simulink model "HaloSim"  (R2019b)
settings: Solver=ode45  StartTime=0.0  StopTime=simTime  FixedStep=10^-5  RelTol=1e-4
values from neighbouring files (symbols this model uses):
  a = zeros(2,1)    [init.m]
  b = zeros(2,1)    [init.m]
  c = zeros(2,1)    [init.m]
  disturbance = 1    [init.m]
  emulation = delta    (= 0.1)    [init.m]
  Gsc = 1.3608    [init.m]
  h = zeros(2,1)    [init.m]
  K = place(A,G,pole)    [init.m]
  k = 0.1    [init.m]
  L2 = 1.1556    [init.m]
  mu = 0.012149    [init.m]
  Omega = 1.8636    [init.m]
  Omega_z = Omega    (= 1.8636)    [init.m]
  phi = 0    [init.m]
  satValue = inf    [init.m]
  sped = 300000    [init.m]
  srp = 1    [init.m]
  x0 = Seq + [ho1;diffho1]    [init.m]
  zeta = 0.9252    [init.m]
libraries: sdolib x1
settings Model: Creator=mohd-  LastModifiedBy=mohd-

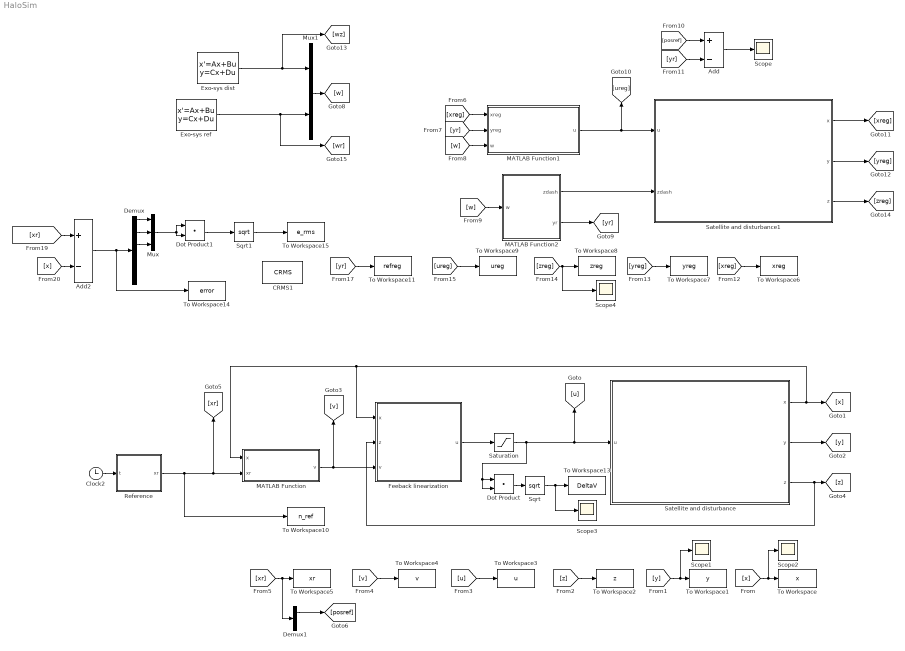
== system HaloSim ==
  Add : Sum  Inputs=+-
  Add2 : Sum  Inputs=+-
  CRMS1 : sdolib/RMS Blocks/CRMS
      settings: SourceProductName=Simulink Design Optimization  SourceProductBaseCode=SO
  Clock2 : Clock
  Demux : Demux  Outputs=6
  Demux1 : Demux  Outputs=[3 3]
  Dot Product : DotProduct  InputSameDT=on  OutDataTypeStr=Inherit: Inherit via internal rule
  Dot Product1 : DotProduct  InputSameDT=on  OutDataTypeStr=Inherit: Inherit via internal rule
  Exo-sys dist : StateSpace  A=[0 -1;1 0]  B=[0;0]  C=eye(2)  D=zeros(2,1)  InitialCondition=[1;0]
  "Exo-sys ref " : StateSpace  A=[0 -Omega;Omega 0]  B=[0;0]  C=eye(2)  D=zeros(2,1)  InitialCondition=[1;0]
  Feeback linearization : MATLAB Function  TreatAsAtomicUnit=on  SystemSampleTime=emulation
  MATLAB Function : MATLAB Function  TreatAsAtomicUnit=on  SystemSampleTime=emulation
  MATLAB Function1 : MATLAB Function  TreatAsAtomicUnit=on  SystemSampleTime=emulation
  MATLAB Function2 : MATLAB Function  TreatAsAtomicUnit=on
  Mux : Mux  Inputs=3
  Mux1 : Mux  Inputs=2
  Reference : MATLAB Function  TreatAsAtomicUnit=on
  Satellite and disturbance : Subsystem
  Satellite and disturbance1 : Subsystem
  Saturation : Saturate  UpperLimit=satValue  LowerLimit=-satValue
  Scope{,1..4} (5 alike) : Scope
  Sqrt : Sqrt  SaturateOnIntegerOverflow=on
  Sqrt1 : Sqrt  SaturateOnIntegerOverflow=on
  To Workspace : ToWorkspace  VariableName=x  SampleTime=10^-3
  To Workspace1 : ToWorkspace  VariableName=y  SampleTime=10^-3
  To Workspace10 : ToWorkspace  VariableName=n_ref  SampleTime=10^-3
  To Workspace11 : ToWorkspace  VariableName=refreg  SampleTime=10^-3
  To Workspace13 : ToWorkspace  VariableName=DeltaV  SampleTime=10^-3
  To Workspace14 : ToWorkspace  VariableName=error  SampleTime=10^-3
  To Workspace15 : ToWorkspace  VariableName=e_rms  SampleTime=10^-3
  To Workspace2 : ToWorkspace  VariableName=z  SampleTime=10^-3
  To Workspace3 : ToWorkspace  VariableName=u  SampleTime=10^-3
  To Workspace4 : ToWorkspace  VariableName=v  SampleTime=10^-3
  To Workspace5 : ToWorkspace  VariableName=xr  SampleTime=10^-3
  To Workspace6 : ToWorkspace  VariableName=xreg  SampleTime=10^-3
  To Workspace7 : ToWorkspace  VariableName=yreg  SampleTime=10^-3
  To Workspace8 : ToWorkspace  VariableName=zreg  SampleTime=10^-3
  To Workspace9 : ToWorkspace  VariableName=ureg  SampleTime=10^-3
  wires:
  Clock2/1 -> Reference/1(t)
  Satellite and disturbance/1(x) -> Feeback linearization/1(x), MATLAB Function/1(x), [x]
  Satellite and disturbance/2(y) -> [y]
  Satellite and disturbance/3(z) -> Feeback linearization/2(z), [z]
  MATLAB Function/1(v) -> Feeback linearization/3(v), [v]
  Reference/1(xr) -> To Workspace10/1, [xr], MATLAB Function/2(xr)
  [x] -> Scope2/1, To Workspace/1
  [y] -> Scope1/1, To Workspace1/1
  [z] -> To Workspace2/1
  [u] -> To Workspace3/1
  [v] -> To Workspace4/1
  [xr] -> Demux1/1, To Workspace5/1
  [xreg] -> MATLAB Function1/1(xreg)
  [yr] -> MATLAB Function1/2(yreg)
  [w] -> MATLAB Function1/3(w)
  [w] -> MATLAB Function2/1(w)
  MATLAB Function2/1(zdash) -> Satellite and disturbance1/2("zdash ")
  MATLAB Function2/2(yr) -> [yr]
  [posref] -> Add/1
  [yr] -> Add/2
  Add/1 -> Scope/1
  [yr] -> To Workspace11/1
  MATLAB Function1/1(u) -> Satellite and disturbance1/1(u), [ureg]
  [yreg] -> To Workspace7/1
  [xreg] -> To Workspace6/1
  Satellite and disturbance1/2(y) -> [yreg]
  Satellite and disturbance1/1(x) -> [xreg]
  Satellite and disturbance1/3(z) -> [zreg]
  [ureg] -> To Workspace9/1
  [zreg] -> Scope4/1, To Workspace8/1
  Add2/1 -> To Workspace14/1, Demux/1
  [xr] -> Add2/1
  Demux/2 -> Mux/2
  [x] -> Add2/2
  Demux/1 -> Mux/1
  Mux/1 -> Dot Product1/1, Dot Product1/2
  Demux/3 -> Mux/3
  Dot Product/1 -> Sqrt/1
  Feeback linearization/1(u) -> Saturation/1
  Saturation/1 -> Dot Product/2, Dot Product/1, Satellite and disturbance/1(u), [u]
  Sqrt/1 -> To Workspace13/1, Scope3/1
  Dot Product1/1 -> Sqrt1/1
  Sqrt1/1 -> To Workspace15/1
  Demux1/1 -> [posref]
  "Exo-sys ref "/1 -> [wr], Mux1/2
  Exo-sys dist/1 -> [wz], Mux1/1
  Mux1/1 -> [w]

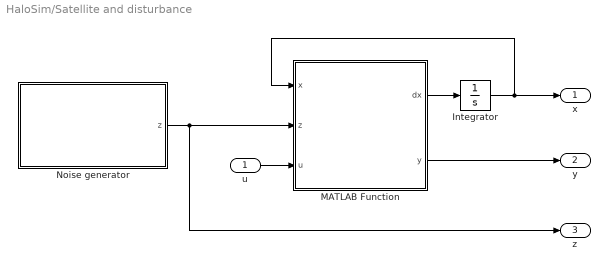
== system HaloSim/Satellite and disturbance ==
  u : Inport
  Integrator : Integrator  InitialCondition=x0
  MATLAB Function : MATLAB Function  TreatAsAtomicUnit=on
  Noise generator : Subsystem
  x : Outport
  y : Outport  Port=2
  z : Outport  Port=3
  wires:
  Integrator/1 -> x/1, MATLAB Function/1(x)
  MATLAB Function/1(dx) -> Integrator/1
  MATLAB Function/2(y) -> y/1
  Noise generator/1(z) -> z/1, MATLAB Function/2(z)
  u/1 -> MATLAB Function/3(u)

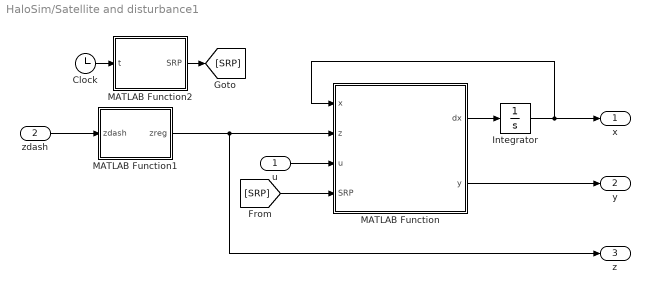
== system HaloSim/Satellite and disturbance1 ==
  u : Inport
  "zdash " : Inport  Port=2
  Clock : Clock
  Integrator : Integrator  InitialCondition=x0
  MATLAB Function : MATLAB Function  TreatAsAtomicUnit=on
  MATLAB Function1 : MATLAB Function  TreatAsAtomicUnit=on
  MATLAB Function2 : MATLAB Function  TreatAsAtomicUnit=on
  x : Outport
  y : Outport  Port=2
  z : Outport  Port=3
  wires:
  Integrator/1 -> x/1, MATLAB Function/1(x)
  MATLAB Function/1(dx) -> Integrator/1
  MATLAB Function/2(y) -> y/1
  "zdash "/1 -> MATLAB Function1/1(zdash)
  u/1 -> MATLAB Function/3(u)
  MATLAB Function1/1(zreg) -> z/1, MATLAB Function/2(z)
  Clock/1 -> MATLAB Function2/1(t)
  MATLAB Function2/1(SRP) -> [SRP]
  [SRP] -> MATLAB Function/4(SRP)

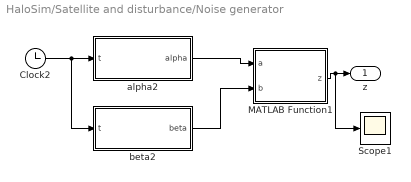
== system HaloSim/Satellite and disturbance/Noise generator ==
  Clock2 : Clock
  MATLAB Function1 : MATLAB Function  TreatAsAtomicUnit=on
  Scope1 : Scope
  alpha2 : MATLAB Function  TreatAsAtomicUnit=on
  beta2 : MATLAB Function  TreatAsAtomicUnit=on
  z : Outport
  wires:
  MATLAB Function1/1(z) -> Scope1/1, z/1
  alpha2/1(alpha) -> MATLAB Function1/1(a)
  beta2/1(beta) -> MATLAB Function1/2(b)
  Clock2/1 -> beta2/1(t), alpha2/1(t)

== matlab function HaloSim/Feeback linearization ==
  data: x input; z input; u output; v input; mu parameter
function u = compensator(x,z,v,mu)
%#codegen


x1 = x(1:3);
x2 = x(4:6);

% M = [-1 0 0;
%     0 -1 0;
%     0 0 0];
% 
% N = [0 -1 0;
%     1 0 0;
%     0 0 0];
% 
% d1r = [-mu - z(4)/(1-mu);0;0];
% d2r = [1-mu + z(4)/mu;0;0];
% 
% ed1 = x1 - d1r;
% absed1 = sqrt(ed1(1)^2+ed1(2)^2+ed1(3)^2);
% ed2 = x1 - d2r;
% absed2 = sqrt(ed2(1)^2+ed2(2)^2+ed2(3)^2);
% 
% f2 = -M*x1 - 2*N*x2 - (2*M*x1 + 2*N*x2)*z(1) ...
%            - M*x1*z(2) - N*x1*z(3) - ed1*(1 - mu)/absed1^3 ...
%            - ed2*mu/absed2^3;
%        
%        
% u = -f2 + v;

% using approx control model

x_1 = x1(1);
x_2 = x1(2);
x_3 = x1(3);
xd_1 = x2(1);
xd_2 = x2(2);

f2 = [x_1 + 2*xd_2 - (mu*(mu + x_1 - 1))/((mu + x_1 - 1)^2 + x_2^2 + x_3^2)^(3/2) + ((mu + x_1)*(mu - 1))/((mu + x_1)^2 + x_2^2 + x_3^2)^(3/2);
    x_2 - 2*xd_1 - (mu*x_2)/((mu + x_1 - 1)^2 + x_2^2 + x_3^2)^(3/2) + (x_2*(mu - 1))/((mu + x_1)^2 + x_2^2 + x_3^2)^(3/2);
    (x_3*(mu - 1))/((mu + x_1)^2 + x_2^2 + x_3^2)^(3/2) - (mu*x_3)/((mu + x_1 - 1)^2 + x_2^2 + x_3^2)^(3/2)];

%F = [f1; f2];

P44 = -2*((x_1+mu)^2+x_2^2+x_3^2)/((x_1+mu)^2+x_2^2+x_3^2)^(5/2) - 2*((x_1-1+mu)^2+x_2^2+x_3^2)/((x_1-1+mu)^2+x_2^2+x_3^2)^(5/2);
P54 = 3*(x_2*(x_1+mu))/((x_1+mu)^2+x_2^2+x_3^2)^(5/2) - 3*(x_2*(x_1-1+mu))/((x_1-1+mu)^2+x_2^2+x_3^2)^(5/2);
P64 = 3*(x_3*(x_1+mu))/((x_1+mu)^2+x_2^2+x_3^2)^(5/2) - 3*x_3*((x_1-1+mu))/((x_1-1+mu)^2+x_2^2+x_3^2)^(5/2);

P = [ 2*x_1 + 2*xd_2, x_1,  x_2, P44;
    2*x_2 - 2*xd_1, x_2, -x_1, P54;
    0,   0,    0, P64];

% F = f2 + [zeros(3,4);P]*z;

u = - f2 - P*z + v;

== matlab function HaloSim/Satellite and disturbance/MATLAB Function ==
  data: x input; z input; dx output; u input; y output; mu parameter
function [dx, y] = Satellite(x,z, u, mu)

x1 = x(1:3);
x2 = x(4:6);

M = [-1 0 0;
    0 -1 0;
    0 0 0];

N = [0 -1 0;
    1 0 0;
    0 0 0];

d1r = [-mu - z(4)/(1-mu);0;0];
d2r = [1-mu + z(4)/mu;0;0];

ed1 = x1 - d1r;
absed1 = sqrt(ed1(1)^2+ed1(2)^2+ed1(3)^2);
ed2 = x1 - d2r;
absed2 = sqrt(ed2(1)^2+ed2(2)^2+ed2(3)^2);

f1 = x2;
f2 = -M*x1 - 2*N*x2 - (2*M*x1 + 2*N*x2)*z(1) ...
           - M*x1*z(2) - N*x1*z(3) - ed1*(1 - mu)/absed1^3 ...
           - ed2*mu/absed2^3;
F = [f1; f2];
G = [zeros(3); eye(3)];


dx = F + G*u;
y  = x1;

== matlab function HaloSim/MATLAB Function ==
  data: x input; v output; xr input; K parameter
function v = linear_control(x, xr, K)

v = -K*(x-xr);

% v = -K*x;

== matlab function HaloSim/MATLAB Function1 ==
  data: xreg input; u output; yreg input; w input; Omega parameter; b parameter; mu parameter; a parameter; e parameter; K parameter; k parameter; c parameter; disturbance parameter; L2 parameter
function u = NLregulator(xreg, yreg, w, Omega, b, mu, a, e, K,k, c, disturbance, L2)
Tz = [b(1)*e 0;0 0;0 -b(1)*e;mu*(1-mu)*a(1)*e 0];
Tr = [k*(1-c(1)+Omega^2)/(2*Omega) 0;0 -k;-k 0];
S2 = [0 -Omega;Omega 0];
Seq = [L2;0;0];
if disturbance == 1
    wz = w(1:2);
else
    wz = zeros(2,1);
end
wr = w(3:4);

pi = [-Tr*wr + Seq;-Tr*S2*wr];

x_1 = pi(1);
x_2 = pi(2);
x_3 = pi(3);
xd_1 = pi(4);
xd_2 = pi(5);

f2 = [x_1 + 2*xd_2 - (mu*(mu + x_1 - 1))/((mu + x_1 - 1)^2 + x_2^2 + x_3^2)^(3/2) + ((mu + x_1)*(mu - 1))/((mu + x_1)^2 + x_2^2 + x_3^2)^(3/2);
    x_2 - 2*xd_1 - (mu*x_2)/((mu + x_1 - 1)^2 + x_2^2 + x_3^2)^(3/2) + (x_2*(mu - 1))/((mu + x_1)^2 + x_2^2 + x_3^2)^(3/2);
    (x_3*(mu - 1))/((mu + x_1)^2 + x_2^2 + x_3^2)^(3/2) - (mu*x_3)/((mu + x_1 - 1)^2 + x_2^2 + x_3^2)^(3/2)];

%F = [f1; f2];

P44 = -2*((x_1+mu)^2+x_2^2+x_3^2)/((x_1+mu)^2+x_2^2+x_3^2)^(5/2) - 2*((x_1-1+mu)^2+x_2^2+x_3^2)/((x_1-1+mu)^2+x_2^2+x_3^2)^(5/2);
P54 = 3*(x_2*(x_1+mu))/((x_1+mu)^2+x_2^2+x_3^2)^(5/2) - 3*(x_2*(x_1-1+mu))/((x_1-1+mu)^2+x_2^2+x_3^2)^(5/2);
P64 = 3*(x_3*(x_1+mu))/((x_1+mu)^2+x_2^2+x_3^2)^(5/2) - 3*x_3*((x_1-1+mu))/((x_1-1+mu)^2+x_2^2+x_3^2)^(5/2);

P = [ 2*x_1 + 2*xd_2, x_1,  x_2, P44;
    2*x_2 - 2*xd_1, x_2, -x_1, P54;
    0,   0,    0, P64];

u = - f2 - P*Tz*wz - Tr*S2^2*wr - K*(xreg-pi);

== matlab function HaloSim/Reference ==
  data: t input; xr output; c parameter; Omega parameter; Omega_z parameter; L2 parameter; k parameter; h parameter; phi parameter; e parameter
function xr = refer(t,c,Omega,Omega_z,L2,k,h, phi,e)
%#codegen
%% modify reference in future to account for Lyapunov orbits

Seq = [L2;0;0;0;0;0];
ho1 = [(-k*(1-c(1)+Omega^2)/(2*Omega))*cos(Omega*t);
       k*sin(Omega*t);
       k*cos(Omega_z*t)];
   
diffho1 = [(k*(1-c(1)+Omega^2)/2)*sin(Omega*t);
           Omega*k*cos(Omega*t);
           -Omega_z*k*sin(Omega_z*t)];
     

       

xr = Seq + [ho1;diffho1];
end

== matlab function HaloSim/Satellite and disturbance1/MATLAB Function1 ==
  data: zdash input; zreg output; disturbance parameter
function zreg = fcn(zdash, disturbance)

if disturbance == 1 
    zreg = zdash;
else
    zreg = zeros(4,1);
end

== matlab function HaloSim/MATLAB Function2 ==
  data: zdash output; w input; yr output; c parameter; Omega parameter; k parameter; a parameter; b parameter; mu parameter; e parameter; L2 parameter
function [zdash,yr] = fcn(w, c, Omega, k, a, b, mu, e, L2)

Seq = [L2;0;0];

T1 = [b(1)*e 0;0 0;0 -b(1)*e;mu*(1-mu)*a(1)*e 0];
Q1 = [k*(1-c(1)+Omega^2)/(2*Omega) 0;0 -k;-k 0];

zdash = T1*w(1:2);
yr = Q1*w(3:4) + Seq;

== matlab function HaloSim/Satellite and disturbance/Noise generator/beta2 ==
  data: t input; beta output; b parameter; phi parameter; e parameter
function beta = b(t,b,phi,e)
%#codegen
b1 = b(1)*e*cos(t+phi);
bd = -b(1)*e*sin(t+phi);
% 
% beta = [b1 + b(2)*e^2*(1+cos(2*(t+phi)));
%          (1+cos(2*(t+phi)))*e^2*b(1)^2/2;
%          bd - 2*b(2)*e^2*sin(2*(t+phi))];

beta = [b1;0;bd];

== matlab function HaloSim/Satellite and disturbance/Noise generator/MATLAB Function1 ==
  data: a input; z output; b input; mu parameter; disturbance parameter
function z = z(a,b,mu,disturbance)
%#codegen
if disturbance == 1
    z = [b;mu*(1-mu)*a];
else
    z = zeros(4,1);
end

== matlab function HaloSim/Satellite and disturbance/Noise generator/alpha2 ==
  data: t input; alpha output; a parameter; phi parameter; e parameter
function alpha = a(t,a,phi,e)
%#codegen
a1 = a(1)*e*cos(t+phi);

% alpha = a1 + a(2)*e^2*(1+cos(2*(t+phi)));
alpha = a1;

== matlab function HaloSim/Satellite and disturbance1/MATLAB Function ==
  data: x input; z input; dx output; u input; y output; mu parameter; SRP input
function [dx, y] = Satellite(x,z, u, mu, SRP)

x1 = x(1:3);
x2 = x(4:6);

M = [-1 0 0;
    0 -1 0;
    0 0 0];

N = [0 -1 0;
    1 0 0;
    0 0 0];

d1r = [-mu - z(4)/(1-mu);0;0];
d2r = [1-mu + z(4)/mu;0;0];

ed1 = x1 - d1r;
absed1 = sqrt(ed1(1)^2+ed1(2)^2+ed1(3)^2);
ed2 = x1 - d2r;
absed2 = sqrt(ed2(1)^2+ed2(2)^2+ed2(3)^2);

f1 = x2;
f2 = -M*x1 - 2*N*x2 - (2*M*x1 + 2*N*x2)*z(1) ...
           - M*x1*z(2) - N*x1*z(3) - ed1*(1 - mu)/absed1^3 ...
           - ed2*mu/absed2^3;
F = [f1; f2 + SRP];
G = [zeros(3); eye(3)];


dx = F + G*u;
y  = x1;

== matlab function HaloSim/Satellite and disturbance1/MATLAB Function2 ==
  data: SRP output; srp parameter; Gsc parameter; sped parameter; zeta parameter; t input
function SRP = fcn(srp, Gsc, sped, zeta,t)

if srp == 1
    SRP = [(Gsc/sped)*(cos(zeta*t))^2;(Gsc/sped)*(sin(zeta*t))^2;0];
else
    SRP = [0;0;0];
end
